simulink model "Servo_Joint"  (R2018a)
settings: Solver=VariableStepAuto  StartTime=0.0  StopTime=10.0  RelTol=1e-3
libraries: simulink x1
settings Model: Creator=Administrator  LastModifiedBy=Administrator

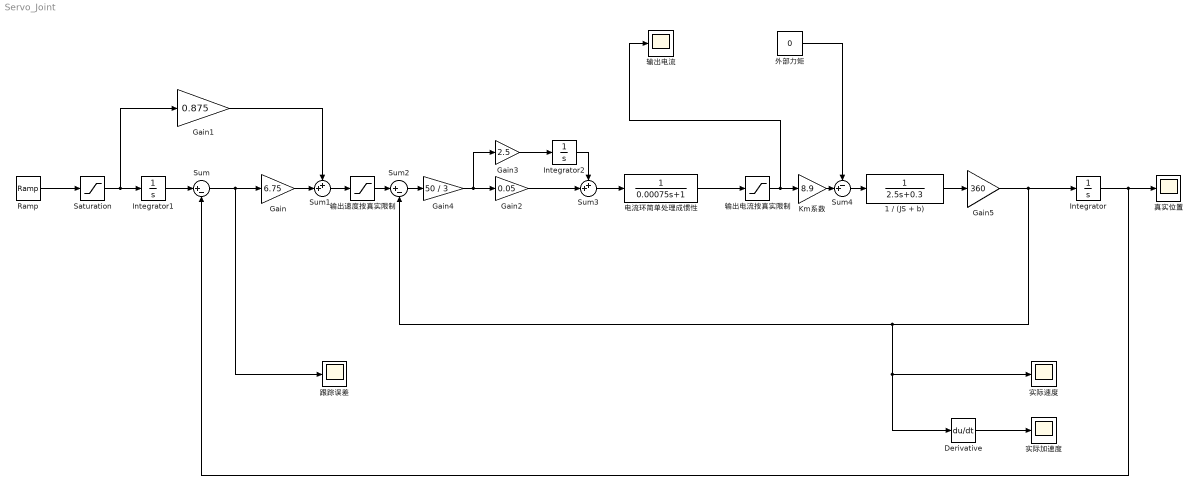
== system Servo_Joint ==
  1 / (JS + b) : TransferFcn  Denominator=[2.5 0.3]
  Derivative : Derivative
  Gain : Gain  Gain=6.75
  Gain1 : Gain  Gain=0.875
  Gain2 : Gain  Gain=0.05
  Gain3 : Gain  Gain=2.5
  Gain4 : Gain  Gain=50 / 3
  Gain5 : Gain  Gain=360
  Integrator : Integrator
  Integrator1 : Integrator
  Integrator2 : Integrator
  Km系数 : Gain  Gain=8.9
  Ramp : simulink/Sources/Ramp  slope=180  start=0  InitialOutput=0
  Saturation : Saturate  UpperLimit=180  LowerLimit=-180
  Sum : Sum  Inputs=|+-
  Sum1 : Sum  Inputs=++|
  Sum2 : Sum  Inputs=|+-
  Sum3 : Sum  Inputs=++|
  Sum4 : Sum  Inputs=-+|
  外部力矩 : Constant  Value=0
  实际加速度 : Scope
  实际速度 : Scope
  电流环简单处理成惯性 : TransferFcn  Denominator=[0.00075 1]
  真实位置 : Scope
  跟踪误差 : Scope
  输出电流 : Scope
  输出电流按真实限制 : Saturate  UpperLimit=32.5  LowerLimit=-32.5
  输出速度按真实限制 : Saturate  UpperLimit=180  LowerLimit=-180
  wires:
  Integrator1/1 -> Sum/1
  Sum/1 -> Gain/1, 跟踪误差/1
  Integrator/1 -> 真实位置/1, Sum/2
  Ramp/1 -> Saturation/1
  Gain/1 -> Sum1/2
  Gain3/1 -> Integrator2/1
  Sum2/1 -> Gain4/1
  Gain2/1 -> Sum3/2
  Integrator2/1 -> Sum3/1
  Gain4/1 -> Gain3/1, Gain2/1
  Gain5/1 -> 实际速度/1, Derivative/1, Sum2/2, Integrator/1
  Km系数/1 -> Sum4/2
  外部力矩/1 -> Sum4/1
  1 / (JS + b)/1 -> Gain5/1
  Sum4/1 -> 1 / (JS + b)/1
  输出电流按真实限制/1 -> 输出电流/1, Km系数/1
  Sum1/1 -> 输出速度按真实限制/1
  输出速度按真实限制/1 -> Sum2/1
  Gain1/1 -> Sum1/1
  Saturation/1 -> Gain1/1, Integrator1/1
  Derivative/1 -> 实际加速度/1
  电流环简单处理成惯性/1 -> 输出电流按真实限制/1
  Sum3/1 -> 电流环简单处理成惯性/1
